simulink model "box_wrench"  (R2022b)
settings: Solver=VariableStepAuto  StartTime=0.0  StopTime=inf  RelTol=1e-3
undefined symbols (not defined in the file or in its folder): Duration, ReferencePoint, StartTime
libraries: robotlib x2
settings Model: Creator=marco  LastModifiedBy=marco

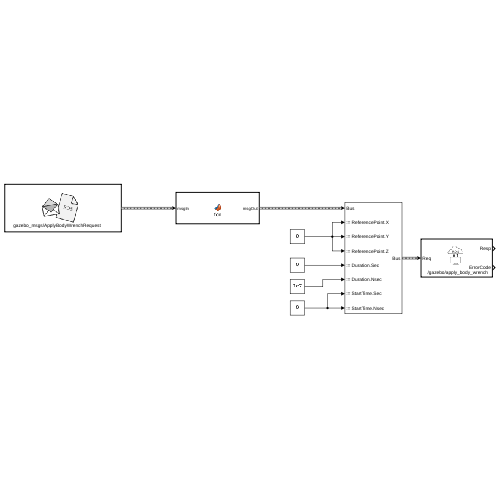
[thumbnail: Simulink's stored preview of the top-level diagram]
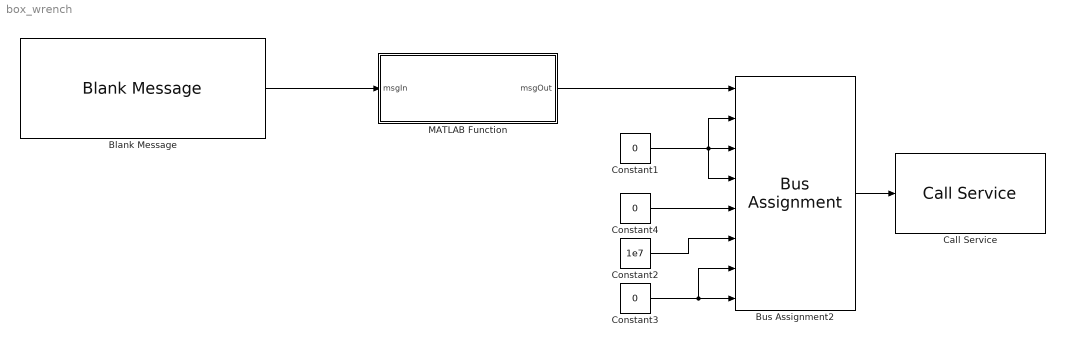
== system box_wrench ==
  Blank Message : robotlib/Blank Message  messageClass=Service Request  entityType=gazebo_msgs/ApplyBodyWrench  messageType=gazebo_msgs/ApplyBodyWrenchRequest  SampleTime=inf  legacyBusStruct=off
      settings: LibrarySourceBlock=roslib/ROS/Blank Message
  Bus Assignment2 : BusAssignment  AssignedSignals=ReferencePoint.X,ReferencePoint.Y,ReferencePoint.Z,Duration.Sec,Duration.Nsec,StartTime.Sec,StartTime.Nsec
  Call Service : robotlib/Call Service  topicSource=Select from ROS network  service=/gazebo/apply_body_wrench  serviceType=gazebo_msgs/ApplyBodyWrench  connectionTimeout=5  keepPersistent=off  ShowErrorCodeOutput=on  legacyBusStruct=off
      settings: LibrarySourceBlock=roslib/ROS/Call Service
  Constant1 : Constant  Value=0
  Constant2 : Constant  Value=1e7
  Constant3 : Constant  Value=0
  Constant4 : Constant  Value=0
  MATLAB Function : MATLAB Function  TreatAsAtomicUnit=on  SystemSampleTime=200
  wires:
  Blank Message/1 -> MATLAB Function/1(msgIn)
  MATLAB Function/1(msgOut) -> Bus Assignment2/1
  Bus Assignment2/1 -> Call Service/1
  Constant2/1 -> Bus Assignment2/6
  Constant1/1 -> Bus Assignment2/3, Bus Assignment2/4, Bus Assignment2/2
  Constant3/1 -> Bus Assignment2/7, Bus Assignment2/8
  Constant4/1 -> Bus Assignment2/5

== matlab function box_wrench/MATLAB Function ==
  data: msgOut output Bus: SL_Bus_box_wrench_gazebo_msgs_ApplyBodyWrenchRequest; msgIn input Bus: SL_Bus_box_wrench_gazebo_msgs_ApplyBodyWrenchRequest
function msgOut  = fcn(msgIn)

msgOut = msgIn;

bodyname = 'box_38_18_14_6::link_0';



lenName = uint32(length(bodyname));
%  msgOut.BodyName = uint8(bodyname);
msgOut.BodyName_SL_Info.CurrentLength = uint32(lenName);


% lenName = uint32(length(bodyname));
msgOut.ReferenceFrame(1:lenName,1) = uint8(bodyname)';
msgOut.ReferenceFrame_SL_Info.CurrentLength = uint32(lenName);

msgOut.BodyName(1:lenName,1) = uint8(convertStringsToChars(bodyname))';


msgOut.Wrench.Force.Y = -50;


% msgOut.Points = msgPoint;
% msgOut.Points.Positions(1:7) = Points(1:7,1);
% msgOut.Points.Positions_SL_Info.CurrentLength = uint32(7);
% 
% msgOut.Points.Velocities(1:7) = [0 ;0 ;0 ;0 ;0 ;0;0];
% msgOut.Points.Velocities_SL_Info.CurrentLength = uint32(7);
% 
% msgOut.Points.Accelerations(1:7) = [0 ;0 ;0 ;0 ;0;0 ;0];
% msgOut.Points.Accelerations_SL_Info.CurrentLength = uint32(7);
% 
% msgOut.Points.Effort(1:7) = [0 ;0 ;0 ;0 ;0 ;0;0];
% msgOut.Points.Effort_SL_Info.CurrentLength = uint32(7);
% 
% msgOut.Header.Stamp.Sec = Time.Sec+1;
% msgOut.Header.Stamp.Nsec = Time.Nsec;
% 
% msgOut.Header.Seq = uint32(0);
% 
% msgOut.Points.TimeFromStart.Sec = 5;
% msgOut.Points.TimeFromStart.Nsec = 0;
% msgOut.Points_SL_Info.CurrentLength = uint32(1);
